simulink model "carSimACCLK"  (Simulink 10.2)
settings: Solver=VariableStepAuto  StartTime=0.0  StopTime=20  FixedStep=1e-3  MaxStep=1e-2  RelTol=1e-3  EnableMultiTasking=on
libraries: simulink x1
settings Model: Creator=hp  LastModifiedBy=11634
settings SolverCC: AlgebraicLoopSolver=LineSearch
settings DataIOCC: LimitDataPoints=on  SignalLoggingName=sigsOut
settings OptimizationCC: ExpressionDepthLimit=2147483647  InitFltsAndDblsToZero=on
settings DebuggingCC: SaveWithParameterizedLinksMsg=none  SignalResolutionControl=TryResolveAllWithWarning  MultiTaskDSMMsg=warning  MultiTaskCondExecSysMsg=none  StateNameClashWarn=warning
settings HardwareCC: TargetUnknown=on
settings GRTTargetCC: TargetFcnLib=ansi_tfl_tmw.mat

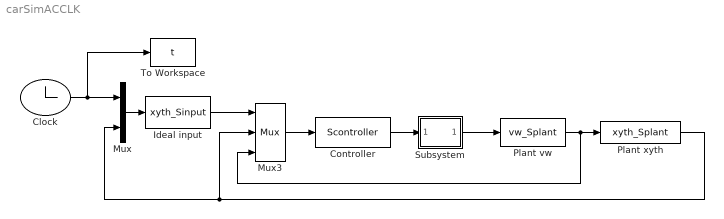
== system carSimACCLK ==
  Clock : Clock
  Controller : S-Function  FunctionName=Scontroller  SFunctionDeploymentMode=off  EnableBusSupport=off
  Ideal input : S-Function  FunctionName=xyth_Sinput  SFunctionDeploymentMode=off  EnableBusSupport=off
  Mux : Mux  Inputs=2
  Mux3 : Mux  Inputs=3
  Plant vw : S-Function  FunctionName=vw_Splant  SFunctionDeploymentMode=off  EnableBusSupport=off
  Plant xyth : S-Function  FunctionName=xyth_Splant  SFunctionDeploymentMode=off  EnableBusSupport=off
  Subsystem : Subsystem
  To Workspace : ToWorkspace  VariableName=t  SampleTime=-1
  wires:
  Plant xyth/1 -> Mux3/2, Mux/2
  Clock/1 -> To Workspace/1, Mux/1
  Mux3/1 -> Controller/1
  Ideal input/1 -> Mux3/1
  Controller/1 -> Subsystem/1(In1)
  Plant vw/1 -> Mux3/3, Plant xyth/1
  Subsystem/1(Out1) -> Plant vw/1
  Mux/1 -> Ideal input/1

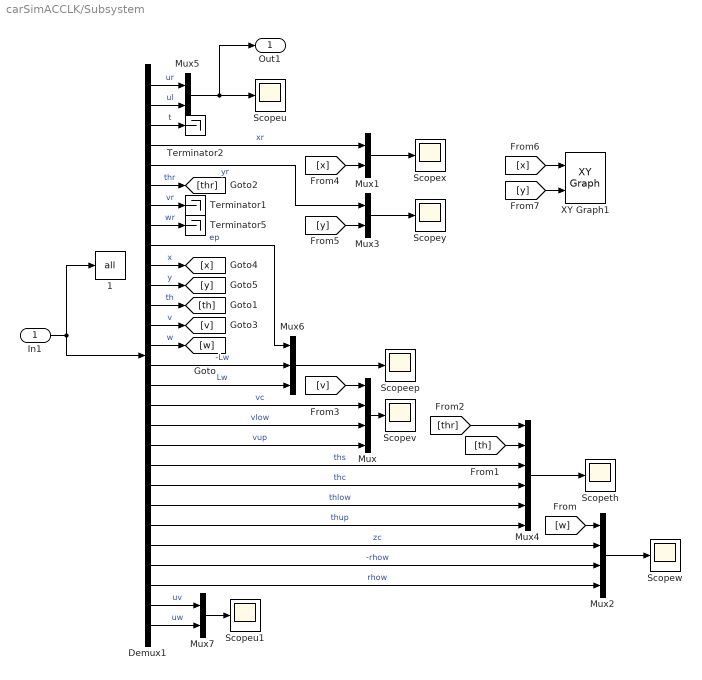
== system carSimACCLK/Subsystem ==
  In1 : Inport
  " 1" : ToWorkspace  VariableName=all  SampleTime=-1
  Demux1 : Demux  Outputs=28
  Mux : Mux
  Mux{1,3,5,7} (4 alike) : Mux  Inputs=2
  Mux2 : Mux
  Mux4 : Mux  Inputs=6
  Mux6 : Mux  Inputs=3
  Scopeep : Scope
  Scopeth : Scope
  Scopeu : Scope
  Scopeu1 : Scope
  Scopev : Scope
  Scopew : Scope
  Scopex : Scope
  Scopey : Scope
  Terminator1 : Terminator
  Terminator2 : Terminator
  Terminator5 : Terminator
  XY Graph1 : simulink/Sinks/XY Graph  xmin=-4  xmax=4  ymin=-4  ymax=4  st=-1
  Out1 : Outport
  wires:
  In1/1 -> " 1"/1, Demux1/1
  Demux1/2 -> Mux5/2  "ul"
  Mux5/1 -> Scopeu/1, Out1/1
  Demux1/1 -> Mux5/1  "ur"
  Demux1/17 -> Mux/2  "vc"
  Demux1/18 -> Mux/3  "vlow"
  Demux1/19 -> Mux/4  "vup"
  Demux1/23 -> Mux4/6  "thup"
  Demux1/22 -> Mux4/5  "thlow"
  Mux2/1 -> Scopew/1
  Mux/1 -> Scopev/1
  Mux4/1 -> Scopeth/1
  Mux3/1 -> Scopey/1
  Mux1/1 -> Scopex/1
  Demux1/26 -> Mux2/4  "rhow"
  Demux1/25 -> Mux2/3  "-rhow"
  Demux1/24 -> Mux2/2  "zc"
  [w] -> Mux2/1
  Demux1/21 -> Mux4/4  "thc"
  Demux1/20 -> Mux4/3  "ths"
  [th] -> Mux4/2
  [thr] -> Mux4/1
  [v] -> Mux/1
  Mux6/1 -> Scopeep/1
  Demux1/16 -> Mux6/3  "Lw"
  Demux1/15 -> Mux6/2  "-Lw"
  Demux1/9 -> Mux6/1  "ep"
  Demux1/14 -> [w]  "w"
  Demux1/13 -> [v]  "v"
  Demux1/12 -> [th]  "th"
  Demux1/6 -> [thr]  "thr"
  Demux1/8 -> Terminator5/1  "wr"
  Demux1/7 -> Terminator1/1  "vr"
  Demux1/3 -> Terminator2/1  "t"
  Demux1/4 -> Mux1/1  "xr"
  Demux1/5 -> Mux3/1  "yr"
  Demux1/10 -> [x]  "x"
  Demux1/11 -> [y]  "y"
  [x] -> Mux1/2
  [y] -> Mux3/2
  [x] -> XY Graph1/1
  [y] -> XY Graph1/2
  Demux1/27 -> Mux7/1  "uv"
  Demux1/28 -> Mux7/2  "uw"
  Mux7/1 -> Scopeu1/1
